simulink model "z3 (1)"  (R2017b)
settings: Solver=FixedStepDiscrete  StartTime=0.0  StopTime=0.0  RelTol=1e-3
libraries: CPOiS_SourcesSinks x8, CPOiS_DataManipulation x3
settings Model: Creator=alis  LastModifiedBy=alis

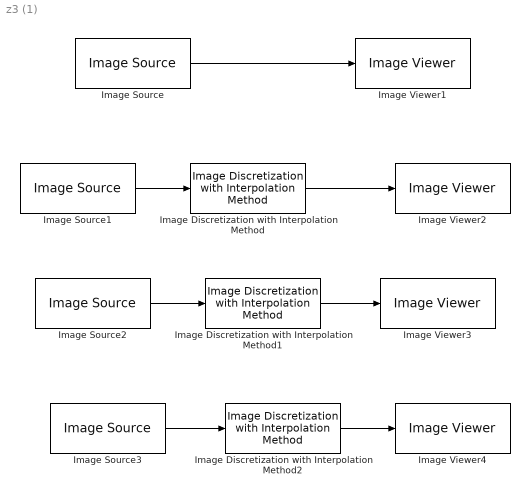
== system z3 (1) ==
  Image Discretization with Interpolation Method : CPOiS_DataManipulation/Image Discretization with Interpolation Method  factor=8  method=nearest
      settings: SourceProductName=CPOiS - Digital image and signal processing
  Image Discretization with Interpolation Method1 : CPOiS_DataManipulation/Image Discretization with Interpolation Method  factor=8  method=bilinear
      settings: SourceProductName=CPOiS - Digital image and signal processing
  Image Discretization with Interpolation Method2 : CPOiS_DataManipulation/Image Discretization with Interpolation Method  factor=8  method=bicubic
      settings: SourceProductName=CPOiS - Digital image and signal processing
  Image Source{,1..3} (4 alike) : CPOiS_SourcesSinks/Image Source  FileSelection=gull.png
      settings: SourceProductName=CPOiS - Digital image and signal processing
  Image Viewer{1..4} (4 alike) : CPOiS_SourcesSinks/Image Viewer
      settings: SourceProductName=CPOiS - Digital image and signal processing
  wires:
  Image Source1/1 -> Image Discretization with Interpolation Method/1
  Image Source/1 -> Image Viewer1/1
  Image Source2/1 -> Image Discretization with Interpolation Method1/1
  Image Source3/1 -> Image Discretization with Interpolation Method2/1
  Image Discretization with Interpolation Method/1 -> Image Viewer2/1
  Image Discretization with Interpolation Method1/1 -> Image Viewer3/1
  Image Discretization with Interpolation Method2/1 -> Image Viewer4/1
